simulink model "pid_altitude_pos"  (R2020b)
settings: Solver=VariableStepAuto  StartTime=0.0  StopTime=10.0  RelTol=1e-3
settings Model: Creator=Théo  LastModifiedBy=Théo

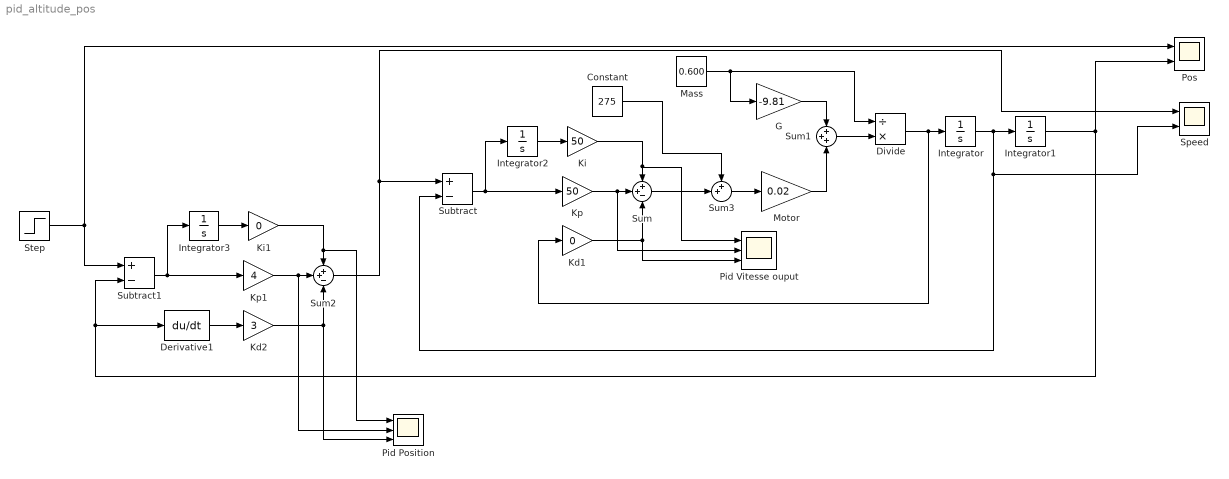
== system pid_altitude_pos ==
  Constant : Constant  Value=275
  Derivative1 : Derivative
  Divide : Product  Inputs=/*
  G : Gain  Gain=-9.81
  Integrator{,1..3} (4 alike) : Integrator
  Kd1 : Gain  Gain=0
  Kd2 : Gain  Gain=3
  Ki : Gain  Gain=50
  Ki1 : Gain  Gain=0
  Kp : Gain  Gain=50
  Kp1 : Gain  Gain=4
  Mass : Constant  Value=0.600
  Motor : Gain  Gain=0.02
  Pid Position : Scope  NumInputPorts=3
  Pid Vitesse ouput : Scope  NumInputPorts=3
  "Pos " : Scope  NumInputPorts=2
  Speed : Scope  NumInputPorts=2
  Step : Step  Time=5  SampleTime=0
  Subtract : Sum  Inputs=+-
  Subtract1 : Sum  Inputs=+-
  Sum : Sum  Inputs=++-
  Sum1 : Sum  Inputs=+++
  Sum2 : Sum  Inputs=++-
  Sum3 : Sum  Inputs=++|
  wires:
  Integrator/1 -> Speed/2, Subtract/2, Integrator1/1
  Divide/1 -> Kd1/1, Integrator/1
  Mass/1 -> G/1, Divide/1
  Subtract/1 -> Kp/1, Integrator2/1
  Sum1/1 -> Divide/2
  Motor/1 -> Sum1/3
  Kd1/1 -> Pid Vitesse ouput/3, Sum/3
  Kp/1 -> Sum/2, Pid Vitesse ouput/2
  Integrator2/1 -> Ki/1
  Ki/1 -> Pid Vitesse ouput/1, Sum/1
  G/1 -> Sum1/1
  Constant/1 -> Sum3/1
  Sum3/1 -> Motor/1
  Sum/1 -> Sum3/2
  Integrator1/1 -> Subtract1/2, Derivative1/1, "Pos "/2
  Sum2/1 -> Speed/1, Subtract/1
  Integrator3/1 -> Ki1/1
  Kd2/1 -> Pid Position/3, Sum2/3
  Ki1/1 -> Pid Position/1, Sum2/1
  Derivative1/1 -> Kd2/1
  Subtract1/1 -> Kp1/1, Integrator3/1
  Kp1/1 -> Pid Position/2, Sum2/2
  Step/1 -> Subtract1/1, "Pos "/1
